simulink model "Turbo_Boostcontrol"  (R2013b)
settings: Solver=ode45  StartTime=0.0  StopTime=10.0  RelTol=1e-3
values from neighbouring files (symbols this model uses):
  A_max_wg = 0.02^2/4*pi    (= 0.000314159265359)    [Project2B.m]
  Cd_wg = 0.9    [Project2B.m]
  dP_thrREF = 10e3    (= 10000)    [Project2B.m]
  KpThr = ??    [Project2B.m]
  KpWg = ?????????    [Project2B.m]
  T_ic = T_im    [Project2B.m]
  TiThr = ??    [Project2B.m]
  TiWg = ?????????    [Project2B.m]
  TqEvsNe =     [TqEvsNeMAP.mat]
  V_ic = 10e-3    (= 0.01)    [Project2B.m]
undefined symbols (not defined in the file or in its folder): etaCmin, etaTmin, gamma_air, Newton, p_amb, R_air, R_exh, Raphson, T_es, V_es
settings Model: Creator=vahne23  LastModifiedBy=vahne23
settings DebuggingCC: SolverPrmCheckMsg=none

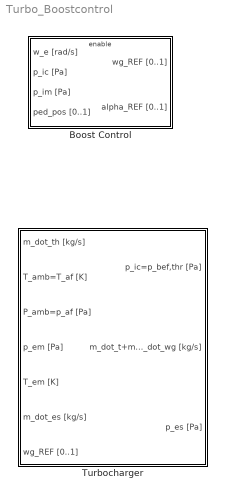
== system Turbo_Boostcontrol ==
  Boost Control : Subsystem
  Turbocharger : Subsystem

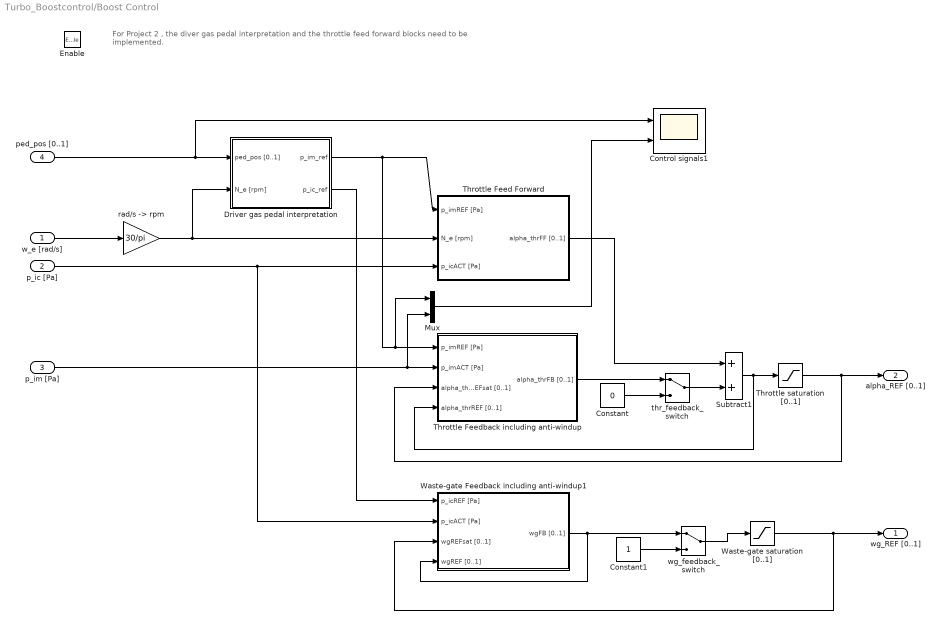
== system Turbo_Boostcontrol/Boost Control ==
  note: For Project 2 , the diver gas pedal interpretation and the throttle feed forward blocks need to be implemented.
  "w_e [rad/s] " : Inport
  p_ic [Pa] : Inport  Port=2
  p_im [Pa] : Inport  Port=3
  ped_pos [0..1] : Inport  Port=4
  Enable : EnablePort
  Constant : Constant  Value=0
  Constant1 : Constant
  Control signals1 : Scope  NumInputPorts=2
      settings: ShowLegends=on  TimeRange=10  YMin=45000~0.2  YMax=85000~0.32  SaveName=ScopeData13  MaxDataPoints=3000
  Driver gas pedal interpretation : Subsystem
  Mux : Mux  Inputs=2
  Subtract1 : Sum
  Throttle saturation [0..1] : Saturate  UpperLimit=1  LowerLimit=0
  "Throttle Feed Forward " : Subsystem
  Throttle Feedback including anti-windup : Subsystem
  Waste-gate saturation [0..1] : Saturate  UpperLimit=1  LowerLimit=0
  Waste-gate Feedback including anti-windup1 : Subsystem
  "rad/s -> rpm" : Gain  Gain=30/pi  SaturateOnIntegerOverflow=on  OutDataTypeStr=Inherit: Same as input  ParamDataTypeStr=Inherit: Same as input
  thr_feedback_switch : ManualSwitch
  wg_feedback_switch : ManualSwitch
  wg_REF [0..1] : Outport
  alpha_REF [0..1] : Outport  Port=2
  wires:
  "Throttle Feed Forward "/1(alpha_thrFF [0..1]) -> Subtract1/1
  Throttle Feedback including anti-windup/1(alpha_thrFB [0..1]) -> thr_feedback_switch/1
  Subtract1/1 -> Throttle saturation [0..1]/1, Throttle Feedback including anti-windup/4(alpha_thrREF [0..1])
  "rad/s -> rpm"/1 -> "Throttle Feed Forward "/2(N_e [rpm]), Driver gas pedal interpretation/2(N_e [rpm])
  Throttle saturation [0..1]/1 -> alpha_REF [0..1]/1, Throttle Feedback including anti-windup/3(alpha_thrREFsat [0..1])
  Waste-gate saturation [0..1]/1 -> Waste-gate Feedback including anti-windup1/3(wgREFsat [0..1]), wg_REF [0..1]/1
  "w_e [rad/s] "/1 -> "rad/s -> rpm"/1
  p_ic [Pa]/1 -> Waste-gate Feedback including anti-windup1/2(p_icACT [Pa]), "Throttle Feed Forward "/3(p_icACT [Pa])
  p_im [Pa]/1 -> Mux/2, Throttle Feedback including anti-windup/2(p_imACT [Pa])
  Driver gas pedal interpretation/1(p_im_ref) -> "Throttle Feed Forward "/1(p_imREF [Pa]), Mux/1, Throttle Feedback including anti-windup/1(p_imREF [Pa])
  Driver gas pedal interpretation/2(p_ic_ref) -> Waste-gate Feedback including anti-windup1/1(p_icREF [Pa])
  Constant/1 -> thr_feedback_switch/2
  thr_feedback_switch/1 -> Subtract1/2
  Mux/1 -> Control signals1/2
  ped_pos [0..1]/1 -> Control signals1/1, Driver gas pedal interpretation/1(ped_pos [0..1])
  Waste-gate Feedback including anti-windup1/1(wgFB [0..1]) -> wg_feedback_switch/1, Waste-gate Feedback including anti-windup1/4(wgREF [0..1])
  Constant1/1 -> wg_feedback_switch/2
  wg_feedback_switch/1 -> Waste-gate saturation [0..1]/1

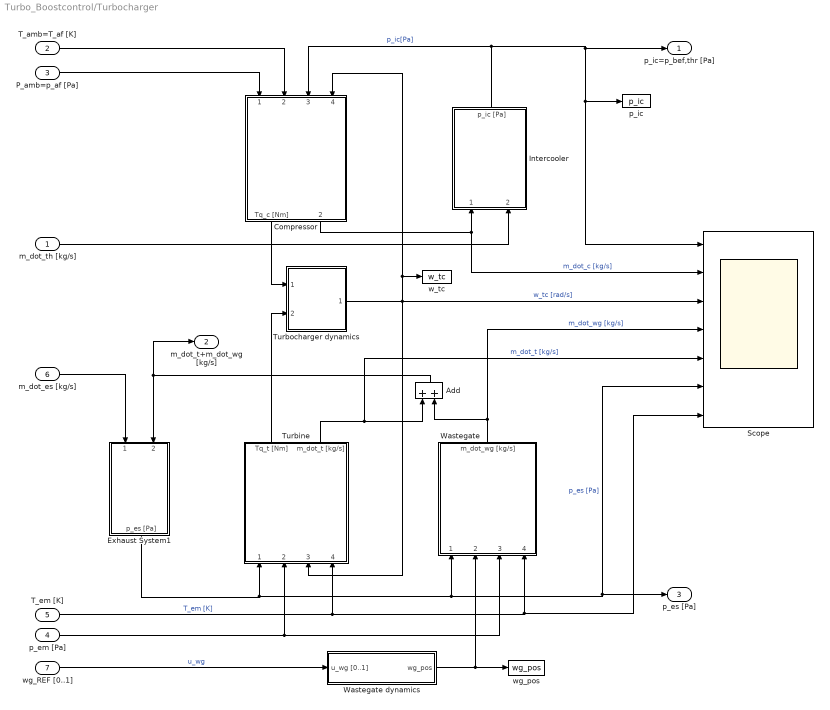
== system Turbo_Boostcontrol/Turbocharger ==
  m_dot_th [kg/s] : Inport
  T_amb=T_af [K] : Inport  Port=2
  "P_amb=p_af [Pa] " : Inport  Port=3
  p_em [Pa] : Inport  Port=4
  T_em [K] : Inport  Port=5
  m_dot_es [kg/s] : Inport  Port=6
  wg_REF [0..1] : Inport  Port=7
  Add : Sum
  Compressor : Subsystem
  Exhaust System1 : Subsystem
  Intercooler : Subsystem
  Scope : Scope  NumInputPorts=7
      settings: ShowLegends=on  TimeRange=60  YMin=100000~-1.73472e-18~2000~-1~0.0025~102500~825  YMax=190000~0.045~12000~1~0.025~103200~1000  SaveName=ScopeData6
  Turbine : Subsystem
  Turbocharger dynamics : Subsystem
  Wastegate : Subsystem
  Wastegate dynamics : Subsystem
  p_ic : ToWorkspace  VariableName=p_ic  SampleTime=-1
  w_tc : ToWorkspace  VariableName=w_tc  SampleTime=-1
  wg_pos : ToWorkspace  VariableName=wg_pos  SampleTime=-1
  p_ic=p_bef,thr [Pa] : Outport
  m_dot_t+m_dot_wg [kg/s] : Outport  Port=2
  p_es [Pa] : Outport  Port=3
  wires:
  Turbocharger dynamics/1(w_tc [rad/s]) -> w_tc/1, Compressor/4(w_tc [rad/s]), Turbine/3(w_tc [rad/s]), Scope/3  "w_tc [rad/s]"
  Wastegate/1(m_dot_wg [kg/s]) -> Scope/4, Add/2  "m_dot_wg [kg/s]"
  Wastegate dynamics/1(wg_pos) -> wg_pos/1, Wastegate/2(wg_pos [0..1])
  wg_REF [0..1]/1 -> Wastegate dynamics/1(u_wg [0..1])  "u_wg"
  Compressor/2(m_dot_c [kg/s]) -> Scope/2, Intercooler/1(Flow in [kg/s])  "m_dot_c [kg/s]"
  Intercooler/1(p_ic [Pa]) -> Compressor/3(p_ic [Pa]), p_ic/1, Scope/1, p_ic=p_bef,thr [Pa]/1  "p_ic[Pa]"
  Compressor/1(Tq_c [Nm]) -> Turbocharger dynamics/1(Tq_c [Nm])
  Turbine/1(Tq_t [Nm]) -> Turbocharger dynamics/2(Tq_t [Nm])
  T_amb=T_af [K]/1 -> Compressor/2(T_af [K])
  "P_amb=p_af [Pa] "/1 -> Compressor/1(p_amb [Pa])
  m_dot_th [kg/s]/1 -> Intercooler/2(Flow  out [kg/s])
  Exhaust System1/1(p_es [Pa]) -> Turbine/1("p_t [Pa] "), Wastegate/1(p_es [Pa]), p_es [Pa]/1, Scope/6  "p_es [Pa]"
  p_em [Pa]/1 -> Turbine/2(p_em [Pa]), Wastegate/3(p_em [Pa])
  Turbine/2(m_dot_t [kg/s]) -> Scope/5, Add/1  "m_dot_t [kg/s]"
  Add/1 -> Exhaust System1/2(Flow in [kg/s]), m_dot_t+m_dot_wg [kg/s]/1
  m_dot_es [kg/s]/1 -> Exhaust System1/1(Flow out [kg/s])
  T_em [K]/1 -> Scope/7, Wastegate/4(T_em [K]), Turbine/4(T_em [k])  "T_em [K]"

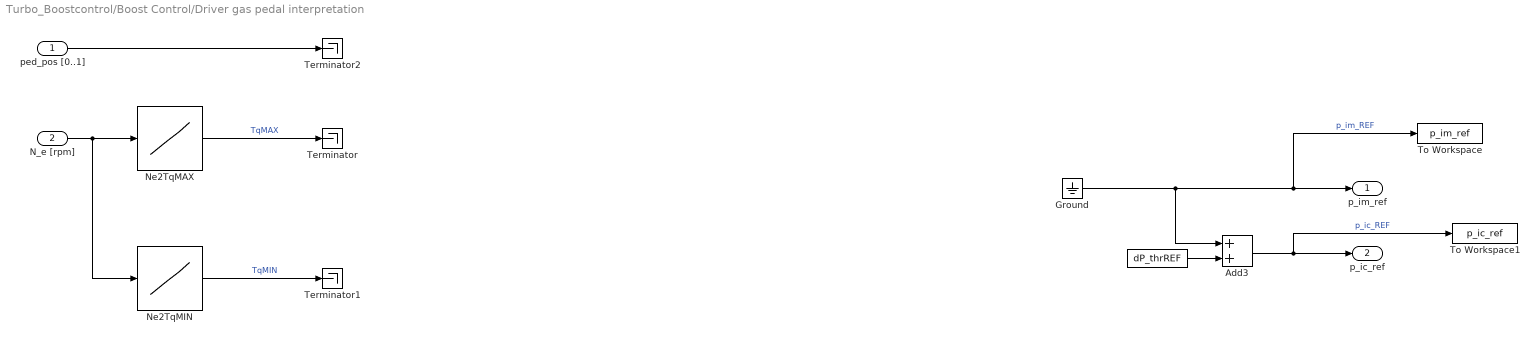
== system Turbo_Boostcontrol/Boost Control/Driver gas pedal interpretation ==
  ped_pos [0..1] : Inport
  N_e [rpm] : Inport  Port=2
  " " : Constant  Value=dP_thrREF
  Add3 : Sum
  Ground : Ground
  Ne2TqMAX : Lookup_n-D  NumberOfTableDimensions=1  BreakpointsForDimension1=TqEvsNe.Ne  Table=TqEvsNe.TqMAX  UseLastTableValue=on  RndMeth=Simplest  InputSameDT=on
  Ne2TqMIN : Lookup_n-D  NumberOfTableDimensions=1  BreakpointsForDimension1=TqEvsNe.Ne  Table=TqEvsNe.TqMIN  UseLastTableValue=on  RndMeth=Simplest  InputSameDT=on
  Terminator : Terminator
  Terminator1 : Terminator
  Terminator2 : Terminator
  To Workspace : ToWorkspace  VariableName=p_im_ref  SampleTime=-1  SaveFormat=Structure With Time
  To Workspace1 : ToWorkspace  VariableName=p_ic_ref  SampleTime=-1  SaveFormat=Structure With Time
  p_im_ref : Outport
  p_ic_ref : Outport  Port=2
  wires:
  N_e [rpm]/1 -> Ne2TqMAX/1, Ne2TqMIN/1
  Ne2TqMIN/1 -> Terminator1/1  "TqMIN"
  Ground/1 -> Add3/1, To Workspace/1, p_im_ref/1  "p_im_REF"
  Add3/1 -> To Workspace1/1, p_ic_ref/1  "p_ic_REF"
  " "/1 -> Add3/2
  Ne2TqMAX/1 -> Terminator/1  "TqMAX"
  ped_pos [0..1]/1 -> Terminator2/1

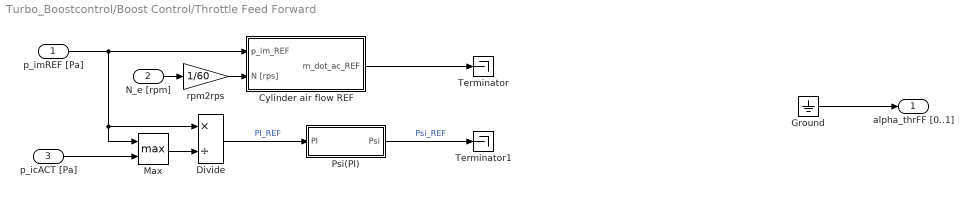
== system Turbo_Boostcontrol/Boost Control/Throttle Feed Forward  ==
  p_imREF [Pa] : Inport
  N_e [rpm] : Inport  Port=2
  p_icACT [Pa] : Inport  Port=3
  Cylinder air flow REF : Subsystem
  Divide : Product  Inputs=*/
  Ground : Ground
  Max : MinMax  Function=max  Inputs=2
  Psi(PI) : Subsystem
  Terminator : Terminator
  Terminator1 : Terminator
  rpm2rps : Gain  Gain=1/60  SaturateOnIntegerOverflow=on  OutDataTypeStr=Inherit: Same as input  ParamDataTypeStr=Inherit: Same as input
  alpha_thrFF [0..1] : Outport
  wires:
  p_imREF [Pa]/1 -> Cylinder air flow REF/1(p_im_REF), Divide/1, Max/1
  N_e [rpm]/1 -> rpm2rps/1
  p_icACT [Pa]/1 -> Max/2
  Cylinder air flow REF/1(m_dot_ac_REF) -> Terminator/1
  Divide/1 -> Psi(PI)/1(PI)  "PI_REF"
  Max/1 -> Divide/2
  rpm2rps/1 -> Cylinder air flow REF/2(N [rps])
  Psi(PI)/1(Psi) -> Terminator1/1  "Psi_REF"
  Ground/1 -> alpha_thrFF [0..1]/1

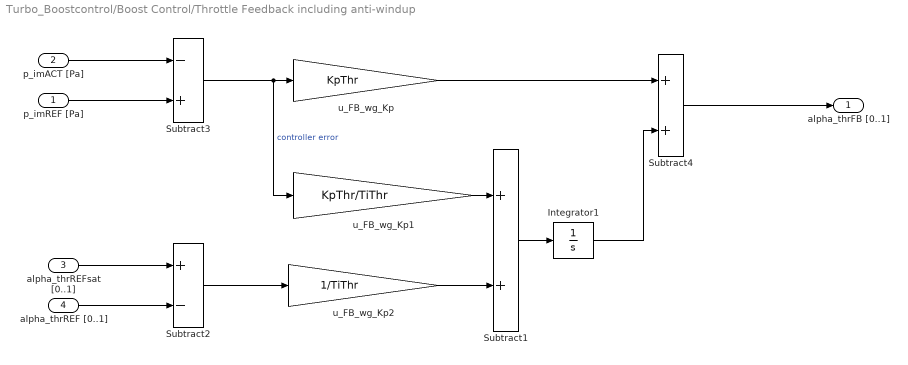
== system Turbo_Boostcontrol/Boost Control/Throttle Feedback including anti-windup ==
  p_imREF [Pa] : Inport
  p_imACT [Pa] : Inport  Port=2
  alpha_thrREFsat [0..1] : Inport  Port=3
  alpha_thrREF [0..1] : Inport  Port=4
  Integrator1 : Integrator  UpperSaturationLimit=5  LowerSaturationLimit=-5
  Subtract1 : Sum
  Subtract2 : Sum  Inputs=+-
  Subtract3 : Sum  Inputs=-+
  Subtract4 : Sum
  u_FB_wg_Kp : Gain  Gain=KpThr
  u_FB_wg_Kp1 : Gain  Gain=KpThr/TiThr
  u_FB_wg_Kp2 : Gain  Gain=1/TiThr
  alpha_thrFB [0..1] : Outport
  wires:
  p_imACT [Pa]/1 -> Subtract3/1
  p_imREF [Pa]/1 -> Subtract3/2
  Subtract3/1 -> u_FB_wg_Kp/1, u_FB_wg_Kp1/1  "controller error"
  u_FB_wg_Kp/1 -> Subtract4/1
  Subtract4/1 -> alpha_thrFB [0..1]/1
  u_FB_wg_Kp1/1 -> Subtract1/1
  alpha_thrREFsat [0..1]/1 -> Subtract2/1
  alpha_thrREF [0..1]/1 -> Subtract2/2
  Subtract2/1 -> u_FB_wg_Kp2/1
  u_FB_wg_Kp2/1 -> Subtract1/2
  Subtract1/1 -> Integrator1/1
  Integrator1/1 -> Subtract4/2

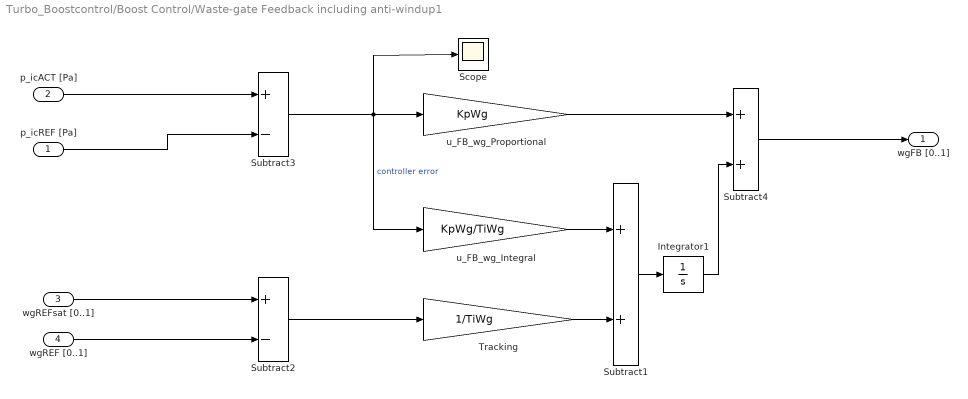
== system Turbo_Boostcontrol/Boost Control/Waste-gate Feedback including anti-windup1 ==
  p_icREF [Pa] : Inport
  p_icACT [Pa] : Inport  Port=2
  wgREFsat [0..1] : Inport  Port=3
  wgREF [0..1] : Inport  Port=4
  Integrator1 : Integrator  InitialCondition=0.3
  Scope : Scope
      settings: YMin=-150000  YMax=100000  SaveName=ScopeData10
  Subtract1 : Sum
  Subtract2 : Sum  Inputs=+-
  Subtract3 : Sum  Inputs=+-
  Subtract4 : Sum
  Tracking : Gain  Gain=1/TiWg
  u_FB_wg_Integral : Gain  Gain=KpWg/TiWg
  u_FB_wg_Proportional : Gain  Gain=KpWg
  wgFB [0..1] : Outport
  wires:
  Integrator1/1 -> Subtract4/2
  Subtract1/1 -> Integrator1/1
  Tracking/1 -> Subtract1/2
  Subtract2/1 -> Tracking/1
  wgREF [0..1]/1 -> Subtract2/2
  wgREFsat [0..1]/1 -> Subtract2/1
  u_FB_wg_Integral/1 -> Subtract1/1
  Subtract4/1 -> wgFB [0..1]/1
  u_FB_wg_Proportional/1 -> Subtract4/1
  Subtract3/1 -> Scope/1, u_FB_wg_Proportional/1, u_FB_wg_Integral/1  "controller error"
  p_icACT [Pa]/1 -> Subtract3/1
  p_icREF [Pa]/1 -> Subtract3/2

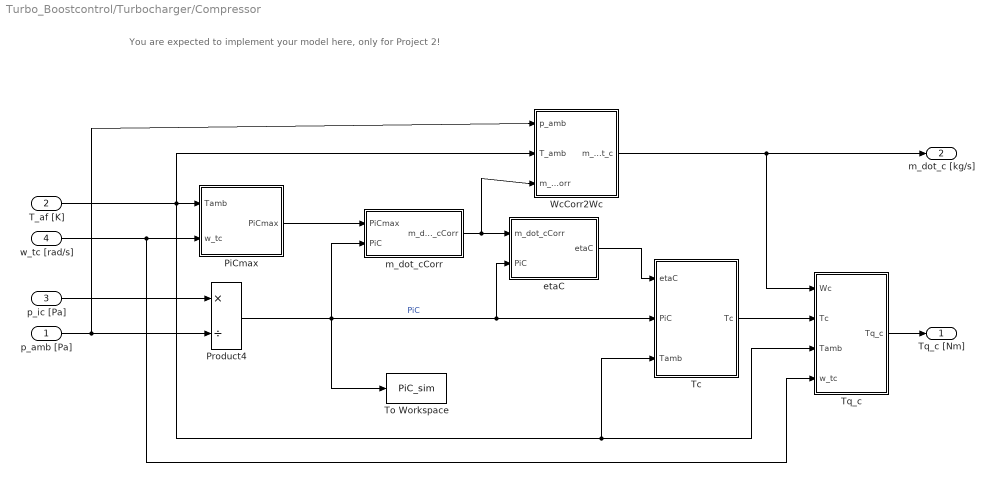
== system Turbo_Boostcontrol/Turbocharger/Compressor ==
  note: You are expected to implement your model here, only for Project 2!
  p_amb [Pa] : Inport
  T_af [K] : Inport  Port=2
  p_ic [Pa] : Inport  Port=3
  w_tc [rad/s] : Inport  Port=4
  PiCmax : Subsystem
  Product4 : Product  Inputs=*/  RndMeth=Zero
  Tc : Subsystem
  To Workspace : ToWorkspace  VariableName=PiC_sim  SampleTime=-1
  Tq_c : Subsystem
  WcCorr2Wc : Subsystem
  etaC : Subsystem
  m_dot_cCorr : Subsystem
  Tq_c [Nm] : Outport
  m_dot_c [kg/s] : Outport  Port=2
  wires:
  w_tc [rad/s]/1 -> PiCmax/2(w_tc), Tq_c/4(w_tc)
  p_ic [Pa]/1 -> Product4/1
  p_amb [Pa]/1 -> WcCorr2Wc/1(p_amb), Product4/2
  T_af [K]/1 -> PiCmax/1(Tamb), WcCorr2Wc/2(T_amb), Tc/3(Tamb), Tq_c/3(Tamb)
  WcCorr2Wc/1(m_dot_c) -> m_dot_c [kg/s]/1, Tq_c/1(Wc)
  Product4/1 -> etaC/2(PiC), Tc/2(PiC), To Workspace/1, m_dot_cCorr/2(PiC)  "PiC"
  PiCmax/1(PiCmax) -> m_dot_cCorr/1(PiCmax)
  m_dot_cCorr/1(m_dot_cCorr) -> WcCorr2Wc/3(m_dot_cCorr), etaC/1(m_dot_cCorr)
  etaC/1(etaC) -> Tc/1(etaC)
  Tc/1(Tc) -> Tq_c/2(Tc)
  Tq_c/1(Tq_c) -> Tq_c [Nm]/1

== system Turbo_Boostcontrol/Turbocharger/Exhaust System1 ==
  Flow out [kg/s] : Inport
  Flow in [kg/s] : Inport  Port=2
  Integrator : Integrator  InitialCondition=103e3
  Product : Product  Inputs=***/  SaturateOnIntegerOverflow=on  OutDataTypeStr=Inherit: Same as first input
  R : Constant  Value=R_exh
  Sum : Sum  Inputs=|+-  SaturateOnIntegerOverflow=on
  T_t : Constant  Value=T_es
  V_es : Constant  Value=V_es
  p_es [Pa] : Outport
  wires:
  V_es/1 -> Product/4
  Sum/1 -> Product/1
  T_t/1 -> Product/3
  R/1 -> Product/2
  Flow out [kg/s]/1 -> Sum/2
  Flow in [kg/s]/1 -> Sum/1
  Product/1 -> Integrator/1
  Integrator/1 -> p_es [Pa]/1

== system Turbo_Boostcontrol/Turbocharger/Intercooler ==
  Flow in [kg/s] : Inport
  Flow  out [kg/s] : Inport  Port=2
  Integrator : Integrator  InitialCondition=p_amb  LowerSaturationLimit=0
  Product : Product  Inputs=***/  SaturateOnIntegerOverflow=on  OutDataTypeStr=Inherit: Same as first input
  R : Constant  Value=R_air
  Sum : Sum  Inputs=|+-  SaturateOnIntegerOverflow=on
  T_ic : Constant  Value=T_ic
  V_ic : Constant  Value=V_ic
  p_ic [Pa] : Outport
  wires:
  Integrator/1 -> p_ic [Pa]/1
  Flow in [kg/s]/1 -> Sum/1
  Flow  out [kg/s]/1 -> Sum/2
  R/1 -> Product/2
  T_ic/1 -> Product/3
  Sum/1 -> Product/1
  V_ic/1 -> Product/4
  Product/1 -> Integrator/1

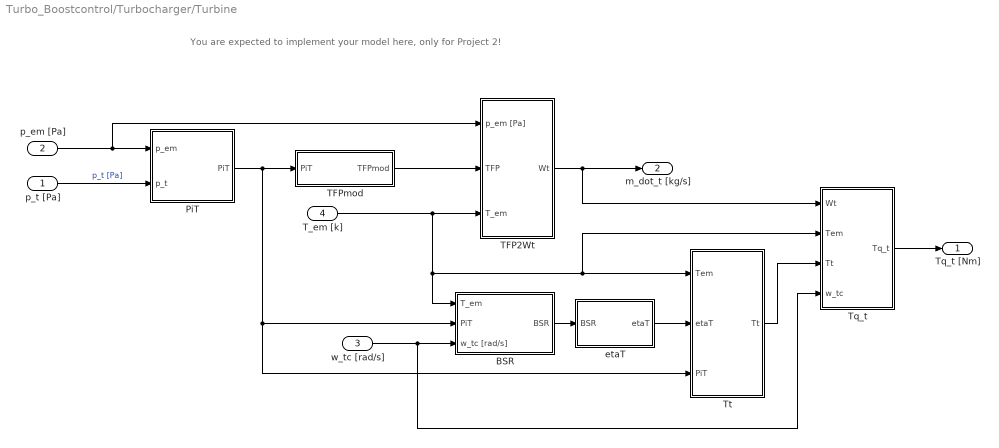
== system Turbo_Boostcontrol/Turbocharger/Turbine ==
  note: You are expected to implement your model here, only for Project 2!
  "p_t [Pa] " : Inport
  p_em [Pa] : Inport  Port=2
  w_tc [rad/s] : Inport  Port=3
  T_em [k] : Inport  Port=4
  BSR : Subsystem
  PiT : Subsystem
  TFP2Wt : Subsystem
  TFPmod : Subsystem
  Tq_t : Subsystem
  Tt : Subsystem
  etaT : Subsystem
  Tq_t [Nm] : Outport
  m_dot_t [kg/s] : Outport  Port=2
  wires:
  w_tc [rad/s]/1 -> BSR/3(w_tc [rad/s]), Tq_t/4(w_tc)
  "p_t [Pa] "/1 -> PiT/2(p_t)  "p_t [Pa]"
  p_em [Pa]/1 -> PiT/1(p_em), TFP2Wt/1(p_em [Pa])
  PiT/1(PiT) -> TFPmod/1(PiT), BSR/2(PiT), Tt/3(PiT)
  TFPmod/1(TFPmod) -> TFP2Wt/2(TFP)
  TFP2Wt/1(Wt) -> m_dot_t [kg/s]/1, Tq_t/1(Wt)
  BSR/1(BSR) -> etaT/1(BSR)
  T_em [k]/1 -> TFP2Wt/3(T_em), BSR/1(T_em), Tq_t/2(Tem), Tt/1(Tem)
  etaT/1(etaT) -> Tt/2(etaT)
  Tt/1(Tt) -> Tq_t/3(Tt)
  Tq_t/1(Tq_t) -> Tq_t [Nm]/1

== system Turbo_Boostcontrol/Turbocharger/Turbocharger dynamics ==
  Tq_c [Nm] : Inport
  Tq_t [Nm] : Inport  Port=2
  Ground : Ground
  Integrator with lower saturation : Integrator  InitialCondition=25e3/30*pi  LimitOutput=on  LowerSaturationLimit="5e3 /  30 * pi"
  Terminator : Terminator
  Terminator1 : Terminator
  w_tc [rad/s] : Outport
  wires:
  Integrator with lower saturation/1 -> w_tc [rad/s]/1
  Ground/1 -> Integrator with lower saturation/1
  Tq_t [Nm]/1 -> Terminator/1
  Tq_c [Nm]/1 -> Terminator1/1

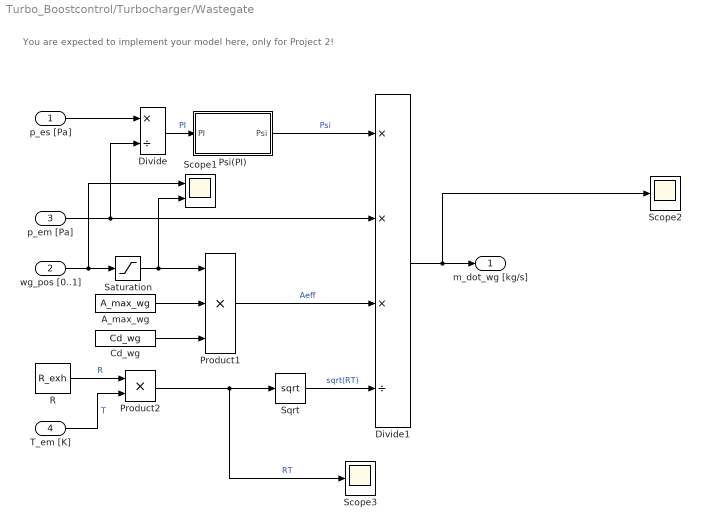
== system Turbo_Boostcontrol/Turbocharger/Wastegate ==
  note: You are expected to implement your model here, only for Project 2!
  p_es [Pa] : Inport
  wg_pos [0..1] : Inport  Port=2
  p_em [Pa] : Inport  Port=3
  T_em [K] : Inport  Port=4
  A_max_wg : Constant  Value=A_max_wg
  Cd_wg : Constant  Value=Cd_wg
  Divide : Product  Inputs=*/
  Divide1 : Product  Inputs=***/
  Product1 : Product  Inputs=3  RndMeth=Zero
  Product2 : Product  RndMeth=Zero
  Psi(PI) : Subsystem
  R : Constant  Value=R_exh
  Saturation : Saturate  UpperLimit=1  LowerLimit=0
  Scope1 : Scope  NumInputPorts=2
      settings: YMin=1~1  YMax=1~1  SaveName=ScopeData3
  Scope2 : Scope
      settings: YMin=0.95  YMax=1.05  SaveName=ScopeData11
  Scope3 : Scope
      settings: YMin=240000  YMax=254000  SaveName=ScopeData12
  Sqrt : Sqrt  AlgorithmType=Newton-Raphson  SaturateOnIntegerOverflow=on
  m_dot_wg [kg/s] : Outport
  wires:
  Divide1/1 -> Scope2/1, m_dot_wg [kg/s]/1
  p_em [Pa]/1 -> Divide/2, Divide1/2
  Divide/1 -> Psi(PI)/1(PI)  "PI"
  Product1/1 -> Divide1/3  "Aeff"
  Product2/1 -> Scope3/1, Sqrt/1  "RT"
  Sqrt/1 -> Divide1/4  "sqrt(RT)"
  Psi(PI)/1(Psi) -> Divide1/1  "Psi"
  R/1 -> Product2/1  "R"
  T_em [K]/1 -> Product2/2  "T"
  wg_pos [0..1]/1 -> Scope1/1, Saturation/1
  A_max_wg/1 -> Product1/2
  Cd_wg/1 -> Product1/3
  Saturation/1 -> Scope1/2, Product1/1
  p_es [Pa]/1 -> Divide/1

== system Turbo_Boostcontrol/Turbocharger/Wastegate dynamics ==
  note: You are expected to implement your model here, only for Project 2!
  u_wg [0..1] : Inport
  Ground : Ground
  Saturation : Saturate  UpperLimit=1  LowerLimit=0
  Terminator : Terminator
  wg_pos : Outport
  wires:
  u_wg [0..1]/1 -> Saturation/1
  Saturation/1 -> Terminator/1
  Ground/1 -> wg_pos/1

== system Turbo_Boostcontrol/Boost Control/Throttle Feed Forward /Cylinder air flow REF ==
  p_im_REF : Inport
  N [rps] : Inport  Port=2
  Ground : Ground
  Terminator : Terminator
  Volymetrisk effektivitet : Subsystem
  m_dot_ac_REF : Outport
  wires:
  p_im_REF/1 -> Volymetrisk effektivitet/1(" p_im")
  N [rps]/1 -> Volymetrisk effektivitet/2(N)
  Volymetrisk effektivitet/1(eta_vol) -> Terminator/1
  Ground/1 -> m_dot_ac_REF/1

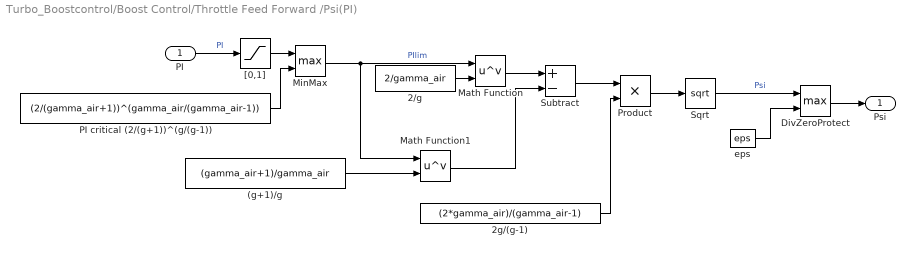
== system Turbo_Boostcontrol/Boost Control/Throttle Feed Forward /Psi(PI) ==
  PI : Inport
  (g+1)/g : Constant  Value=(gamma_air+1)/gamma_air
  2/g : Constant  Value=2/gamma_air
  2g/(g-1) : Constant  Value=(2*gamma_air)/(gamma_air-1)
  DivZeroProtect : MinMax  Function=max  Inputs=2
  Math Function : Math  Operator=pow  SaturateOnIntegerOverflow=on
  Math Function1 : Math  Operator=pow  SaturateOnIntegerOverflow=on
  MinMax : MinMax  Function=max  Inputs=2
  PI critical (2/(g+1))^(g/(g-1)) : Constant  Value=(2/(gamma_air+1))^(gamma_air/(gamma_air-1))
  Product : Product  RndMeth=Zero
  Sqrt : Sqrt  AlgorithmType=Newton-Raphson  SaturateOnIntegerOverflow=on
  Subtract : Sum  Inputs=+-
  "[0,1]" : Saturate  UpperLimit=1  LowerLimit=0
  eps : Constant  Value=eps
  Psi : Outport
  wires:
  PI/1 -> "[0,1]"/1  "PI"
  PI critical (2/(g+1))^(g/(g-1))/1 -> MinMax/2
  MinMax/1 -> Math Function/1, Math Function1/1  "PIlim"
  2/g/1 -> Math Function/2
  (g+1)/g/1 -> Math Function1/2
  "[0,1]"/1 -> MinMax/1
  Math Function/1 -> Subtract/1
  Math Function1/1 -> Subtract/2
  Subtract/1 -> Product/1
  2g/(g-1)/1 -> Product/2
  Product/1 -> Sqrt/1
  Sqrt/1 -> DivZeroProtect/1  "Psi"
  eps/1 -> DivZeroProtect/2
  DivZeroProtect/1 -> Psi/1

== system Turbo_Boostcontrol/Turbocharger/Compressor/PiCmax ==
  Tamb : Inport
  w_tc : Inport  Port=2
  Ground : Ground
  Terminator : Terminator
  Terminator1 : Terminator
  PiCmax : Outport
  wires:
  w_tc/1 -> Terminator/1
  Tamb/1 -> Terminator1/1
  Ground/1 -> PiCmax/1

== system Turbo_Boostcontrol/Turbocharger/Compressor/Tc ==
  etaC : Inport
  PiC : Inport  Port=2
  Tamb : Inport  Port=3
  Ground : Ground
  Terminator : Terminator
  Terminator1 : Terminator
  Terminator2 : Terminator
  Tc : Outport
  wires:
  Tamb/1 -> Terminator2/1
  etaC/1 -> Terminator1/1
  PiC/1 -> Terminator/1
  Ground/1 -> Tc/1

== system Turbo_Boostcontrol/Turbocharger/Compressor/Tq_c ==
  Wc : Inport
  Tc : Inport  Port=2
  Tamb : Inport  Port=3
  w_tc : Inport  Port=4
  Ground : Ground
  Terminator{,1..3} (4 alike) : Terminator
  Tq_c : Outport
  wires:
  Tamb/1 -> Terminator2/1
  Tc/1 -> Terminator1/1
  Ground/1 -> Tq_c/1
  Wc/1 -> Terminator/1
  w_tc/1 -> Terminator3/1

== system Turbo_Boostcontrol/Turbocharger/Compressor/WcCorr2Wc ==
  p_amb : Inport
  T_amb : Inport  Port=2
  m_dot_cCorr : Inport  Port=3
  Ground : Ground
  Terminator : Terminator
  Terminator1 : Terminator
  Terminator2 : Terminator
  m_dot_c : Outport
  wires:
  Ground/1 -> m_dot_c/1
  T_amb/1 -> Terminator2/1
  p_amb/1 -> Terminator1/1
  m_dot_cCorr/1 -> Terminator/1

== system Turbo_Boostcontrol/Turbocharger/Compressor/etaC ==
  m_dot_cCorr : Inport
  PiC : Inport  Port=2
  Ground : Ground
  Max : MinMax  Function=max  Inputs=2
  Terminator : Terminator
  Terminator1 : Terminator
  etaCmin : Constant  Value=etaCmin
  etaC : Outport
  wires:
  Ground/1 -> Max/1
  etaCmin/1 -> Max/2
  Max/1 -> etaC/1
  m_dot_cCorr/1 -> Terminator/1
  PiC/1 -> Terminator1/1

== system Turbo_Boostcontrol/Turbocharger/Compressor/m_dot_cCorr ==
  PiCmax : Inport
  PiC : Inport  Port=2
  Ground : Ground
  Terminator : Terminator
  Terminator1 : Terminator
  To Workspace1 : ToWorkspace  VariableName=m_dot_cCorr  SampleTime=-1
  m_dot_cCorr : Outport
  wires:
  Ground/1 -> To Workspace1/1, m_dot_cCorr/1  "m_dot_cCorr"
  PiCmax/1 -> Terminator/1
  PiC/1 -> Terminator1/1

== system Turbo_Boostcontrol/Turbocharger/Turbine/BSR ==
  T_em : Inport
  PiT : Inport  Port=2
  w_tc [rad/s] : Inport  Port=3
  Ground : Ground
  Terminator : Terminator
  Terminator1 : Terminator
  Terminator2 : Terminator
  BSR : Outport
  wires:
  w_tc [rad/s]/1 -> Terminator/1
  PiT/1 -> Terminator1/1
  T_em/1 -> Terminator2/1
  Ground/1 -> BSR/1

== system Turbo_Boostcontrol/Turbocharger/Turbine/PiT ==
  p_em : Inport
  p_t : Inport  Port=2
  MinMax : MinMax  Function=max  Inputs=2
  Product4 : Product  Inputs=*/  RndMeth=Zero
  one1 : Constant
  PiT : Outport
  wires:
  Product4/1 -> MinMax/1
  one1/1 -> MinMax/2
  p_em/1 -> Product4/1
  MinMax/1 -> PiT/1  "PiT"
  p_t/1 -> Product4/2

== system Turbo_Boostcontrol/Turbocharger/Turbine/TFP2Wt ==
  p_em [Pa] : Inport
  TFP : Inport  Port=2
  T_em : Inport  Port=3
  Ground : Ground
  Terminator : Terminator
  Terminator1 : Terminator
  Terminator2 : Terminator
  Wt : Outport
  wires:
  p_em [Pa]/1 -> Terminator1/1
  T_em/1 -> Terminator2/1
  TFP/1 -> Terminator/1
  Ground/1 -> Wt/1

== system Turbo_Boostcontrol/Turbocharger/Turbine/TFPmod ==
  PiT : Inport
  Ground : Ground
  Terminator : Terminator
  TFPmod : Outport
  wires:
  PiT/1 -> Terminator/1
  Ground/1 -> TFPmod/1

== system Turbo_Boostcontrol/Turbocharger/Turbine/Tq_t ==
  Wt : Inport
  Tem : Inport  Port=2
  Tt : Inport  Port=3
  w_tc : Inport  Port=4
  Ground : Ground
  Terminator{,1..3} (4 alike) : Terminator
  Tq_t : Outport
  wires:
  Ground/1 -> Tq_t/1
  w_tc/1 -> Terminator3/1
  Tt/1 -> Terminator2/1
  Tem/1 -> Terminator1/1
  Wt/1 -> Terminator/1

== system Turbo_Boostcontrol/Turbocharger/Turbine/Tt ==
  Tem : Inport
  etaT : Inport  Port=2
  PiT : Inport  Port=3
  Ground : Ground
  Terminator : Terminator
  Terminator1 : Terminator
  Terminator2 : Terminator
  Tt : Outport
  wires:
  Tem/1 -> Terminator2/1
  etaT/1 -> Terminator1/1
  PiT/1 -> Terminator/1
  Ground/1 -> Tt/1

== system Turbo_Boostcontrol/Turbocharger/Turbine/etaT ==
  BSR : Inport
  Ground : Ground
  Max : MinMax  Function=max  Inputs=2
  Terminator : Terminator
  etaTmin : Constant  Value=etaTmin
  etaT : Outport
  wires:
  Max/1 -> etaT/1
  etaTmin/1 -> Max/2
  BSR/1 -> Terminator/1
  Ground/1 -> Max/1

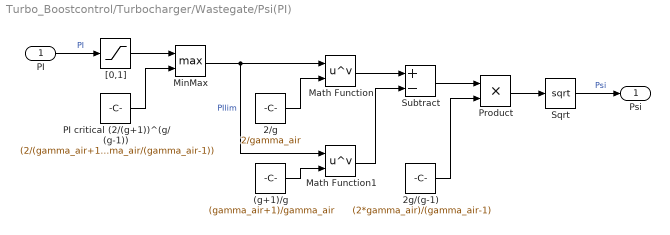
== system Turbo_Boostcontrol/Turbocharger/Wastegate/Psi(PI) ==
  PI : Inport
  (g+1)/g : Constant  Value=(gamma_air+1)/gamma_air
  2/g : Constant  Value=2/gamma_air
  2g/(g-1) : Constant  Value=(2*gamma_air)/(gamma_air-1)
  Math Function : Math  Operator=pow  SaturateOnIntegerOverflow=on
  Math Function1 : Math  Operator=pow  SaturateOnIntegerOverflow=on
  MinMax : MinMax  Function=max  Inputs=2
  PI critical (2/(g+1))^(g/(g-1)) : Constant  Value=(2/(gamma_air+1))^(gamma_air/(gamma_air-1))
  Product : Product  RndMeth=Zero
  Sqrt : Sqrt  AlgorithmType=Newton-Raphson  SaturateOnIntegerOverflow=on
  Subtract : Sum  Inputs=+-
  "[0,1]" : Saturate  UpperLimit=1  LowerLimit=0
  Psi : Outport
  wires:
  PI/1 -> "[0,1]"/1  "PI"
  PI critical (2/(g+1))^(g/(g-1))/1 -> MinMax/2
  MinMax/1 -> Math Function/1, Math Function1/1  "PIlim"
  2/g/1 -> Math Function/2
  (g+1)/g/1 -> Math Function1/2
  "[0,1]"/1 -> MinMax/1
  Math Function/1 -> Subtract/1
  Math Function1/1 -> Subtract/2
  Subtract/1 -> Product/1
  2g/(g-1)/1 -> Product/2
  Product/1 -> Sqrt/1
  Sqrt/1 -> Psi/1  "Psi"

== system Turbo_Boostcontrol/Boost Control/Throttle Feed Forward /Cylinder air flow REF/Volymetrisk effektivitet ==
  " p_im" : Inport
  N : Inport  Port=2
  Ground : Ground
  Terminator : Terminator
  Terminator1 : Terminator
  eta_vol : Outport
  wires:
  N/1 -> Terminator/1
  " p_im"/1 -> Terminator1/1
  Ground/1 -> eta_vol/1
